simulink model "NDS_FSFB"  (R2022b)
settings: Solver=VariableStepAuto  StartTime=0.0  StopTime=100  RelTol=1e-3
values from neighbouring files (symbols this model uses):
  C_LVLH_ECI0 = [xLVLH__ECI'; yLVLH__ECI'; zLVLH__ECI']    [NDS_FSFBmat.m]
  E_b_LVLH0 = quat2EA(q_b_LVLH0)    [NDS_FSFBmat.m]
  J = [Ixx 0 0 ; 0 Iyy 0; 0 0 Izz]    [NDS_FSFBmat.m]
  kd = 2 .* J * DCR .* w_n    [NDS_FSFBmat.m]
  kp = 2 .* J .* (w_n).^2    [NDS_FSFBmat.m]
  mu = 398600    [ECIstate.m]    (also in NDS_FSFBmat.m)
  n = norm(vECI0)/norm(rECI0)    [NDS_FSFBmat.m]
  q_b_LVLH0 = [eps_LVLH_b0; eta_LVLH_b0]    [NDS_FSFBmat.m]
  q_LVLH_b_c = [0 0 0 1]'    [NDS_FSFBmat.m]
  q_LVLH_ECI0 = C2quat(C_LVLH_ECI0)    [NDS_FSFBmat.m]
  w_ECI_b0_b = w_LVLH_b0_b    [NDS_FSFBmat.m]
undefined symbols (not defined in the file or in its folder): rECI0, vECI0, w_b_ECI0_b
libraries: matrix_library x1
settings Model: Creator=nathaliadesouza  LastModifiedBy=nathaliadesouza
settings DataIOCC: DatasetSignalFormat=timetable

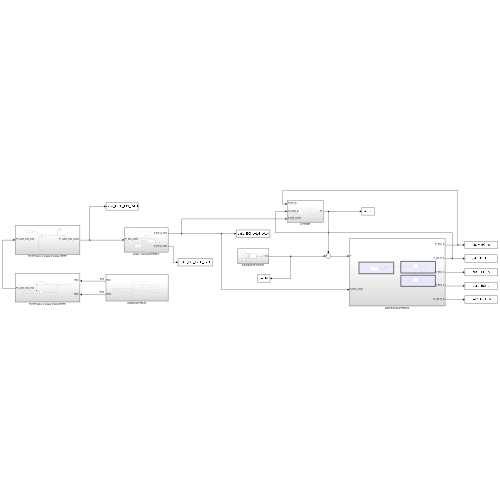
[thumbnail: Simulink's stored preview of the top-level diagram]
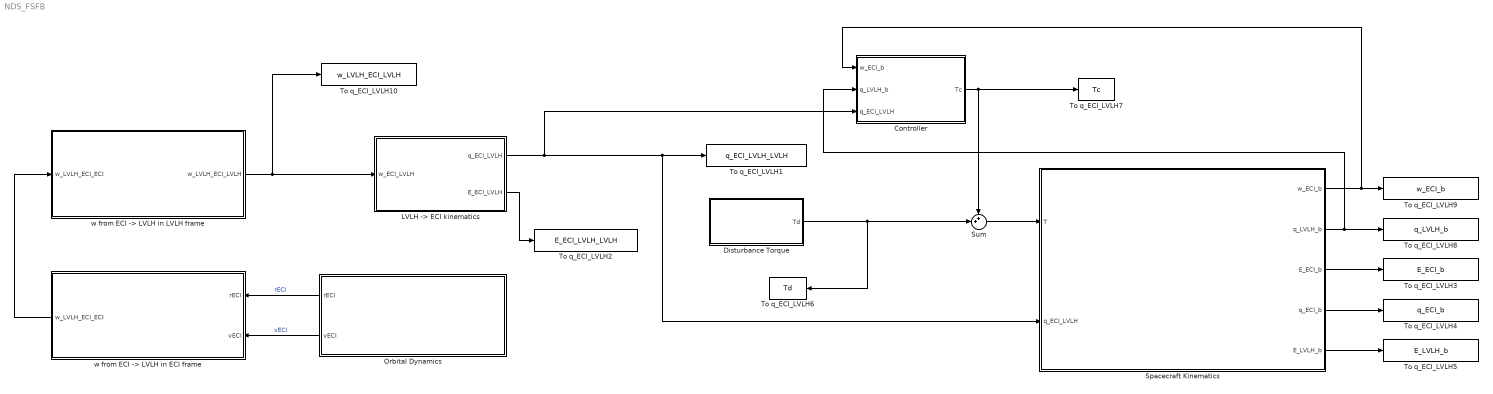
== system NDS_FSFB ==
  Controller : Subsystem
  Disturbance Torque : Subsystem
  "LVLH -> ECI kinematics" : Subsystem
  Orbital Dynamics : Subsystem
  Spacecraft Kinematics : Subsystem
  Sum : Sum  Inputs=++|
  To q_ECI_LVLH1 : ToWorkspace  VariableName=q_ECI_LVLH_LVLH  SaveFormat=Timeseries  SampleTime=-1
  To q_ECI_LVLH10 : ToWorkspace  VariableName=w_LVLH_ECI_LVLH  SaveFormat=Timeseries  SampleTime=-1
  To q_ECI_LVLH2 : ToWorkspace  VariableName=E_ECI_LVLH_LVLH  SaveFormat=Timeseries  SampleTime=-1
  To q_ECI_LVLH3 : ToWorkspace  VariableName=E_ECI_b  SaveFormat=Timeseries  SampleTime=-1
  To q_ECI_LVLH4 : ToWorkspace  VariableName=q_ECI_b  SaveFormat=Timeseries  SampleTime=-1
  To q_ECI_LVLH5 : ToWorkspace  VariableName=E_LVLH_b  SaveFormat=Timeseries  SampleTime=-1
  To q_ECI_LVLH6 : ToWorkspace  VariableName=Td  SaveFormat=Timeseries  SampleTime=-1
  To q_ECI_LVLH7 : ToWorkspace  VariableName=Tc  SaveFormat=Timeseries  SampleTime=-1
  To q_ECI_LVLH8 : ToWorkspace  VariableName=q_LVLH_b  SaveFormat=Timeseries  SampleTime=-1
  To q_ECI_LVLH9 : ToWorkspace  VariableName=w_ECI_b  SaveFormat=Timeseries  SampleTime=-1
  "w from ECI -> LVLH in ECI frame" : Subsystem
  "w from ECI -> LVLH in LVLH frame" : Subsystem
  wires:
  Disturbance Torque/1(Td) -> To q_ECI_LVLH6/1, Sum/2
  "w from ECI -> LVLH in ECI frame"/1(w_LVLH_ECI_ECI) -> "w from ECI -> LVLH in LVLH frame"/1(w_LVLH_ECI_ECI)
  "w from ECI -> LVLH in LVLH frame"/1(w_LVLH_ECI_LVLH) -> To q_ECI_LVLH10/1, "LVLH -> ECI kinematics"/1(w_ECI_LVLH)
  Orbital Dynamics/1(rECI) -> "w from ECI -> LVLH in ECI frame"/1(rECI)  "rECI"
  Orbital Dynamics/2(vECI) -> "w from ECI -> LVLH in ECI frame"/2(vECI)  "vECI"
  "LVLH -> ECI kinematics"/2(E_ECI_LVLH) -> To q_ECI_LVLH2/1
  Sum/1 -> Spacecraft Kinematics/1(T)
  Spacecraft Kinematics/2(q_LVLH_b) -> Controller/2(q_LVLH_b), To q_ECI_LVLH8/1
  Spacecraft Kinematics/1(w_ECI_b) -> Controller/1(w_ECI_b), To q_ECI_LVLH9/1
  Spacecraft Kinematics/3(E_ECI_b) -> To q_ECI_LVLH3/1
  Spacecraft Kinematics/4(q_ECI_b) -> To q_ECI_LVLH4/1
  Spacecraft Kinematics/5(E_LVLH_b) -> To q_ECI_LVLH5/1
  "LVLH -> ECI kinematics"/1(q_ECI_LVLH) -> Spacecraft Kinematics/2(q_ECI_LVLH), To q_ECI_LVLH1/1, Controller/3(q_ECI_LVLH)
  Controller/1(Tc) -> Sum/1, To q_ECI_LVLH7/1

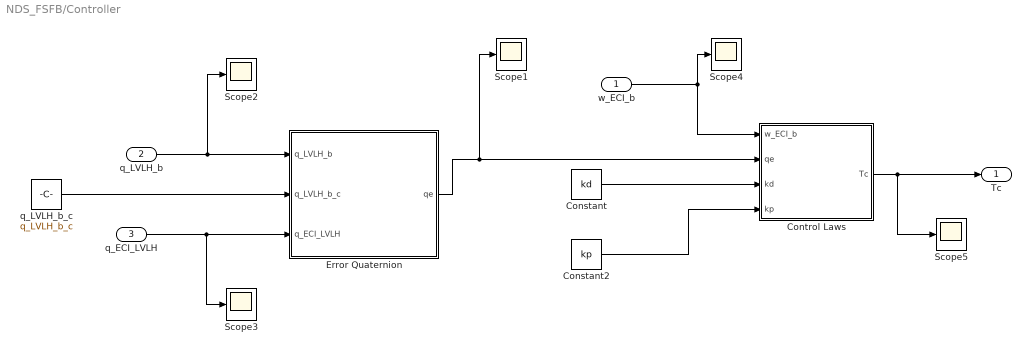
== system NDS_FSFB/Controller ==
  w_ECI_b : Inport
  q_LVLH_b : Inport  Port=2
  q_ECI_LVLH : Inport  Port=3
  Constant : Constant  Value=kd
  Constant2 : Constant  Value=kp
  Control Laws : MATLAB Function  TreatAsAtomicUnit=on
  Error Quaternion : MATLAB Function  TreatAsAtomicUnit=on
  Scope{1..5} (5 alike) : Scope
  q_LVLH_b_c : Constant  Value=q_LVLH_b_c
  Tc : Outport
  wires:
  q_LVLH_b_c/1 -> Error Quaternion/2(q_LVLH_b_c)
  Constant/1 -> Control Laws/3(kd)
  q_LVLH_b/1 -> Scope2/1, Error Quaternion/1(q_LVLH_b)
  q_ECI_LVLH/1 -> Scope3/1, Error Quaternion/3(q_ECI_LVLH)
  Error Quaternion/1(qe) -> Scope1/1, Control Laws/2(qe)
  Constant2/1 -> Control Laws/4(kp)
  w_ECI_b/1 -> Scope4/1, Control Laws/1(w_ECI_b)
  Control Laws/1(Tc) -> Scope5/1, Tc/1

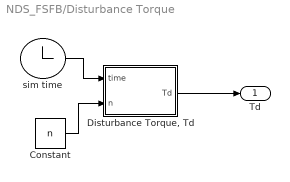
== system NDS_FSFB/Disturbance Torque ==
  Constant : Constant  Value=n
  "Disturbance Torque, Td" : MATLAB Function  TreatAsAtomicUnit=on
  sim time : Clock
  Td : Outport
  wires:
  "Disturbance Torque, Td"/1(Td) -> Td/1
  sim time/1 -> "Disturbance Torque, Td"/1(time)
  Constant/1 -> "Disturbance Torque, Td"/2(n)

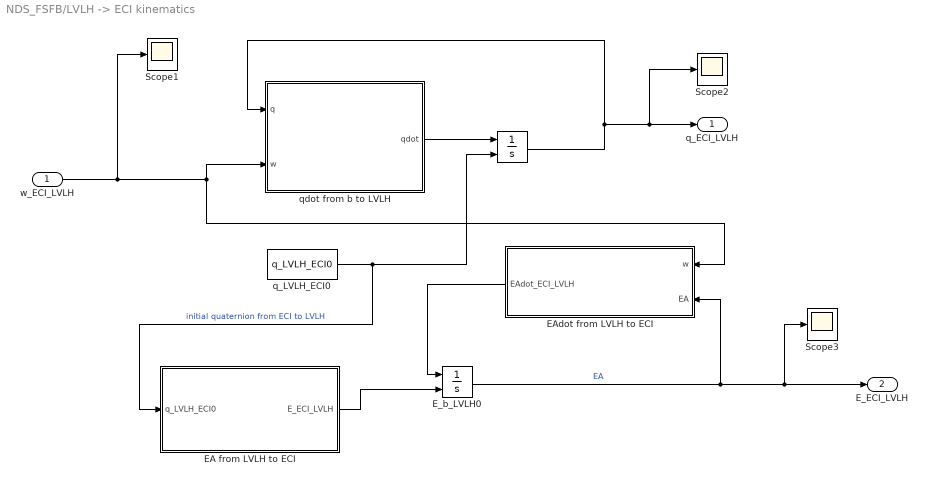
== system NDS_FSFB/LVLH -> ECI kinematics ==
  w_ECI_LVLH : Inport
  " " : Integrator  InitialConditionSource=external  InitialCondition=q_b_LVLH0
  EA from LVLH to ECI : MATLAB Function  TreatAsAtomicUnit=on
  EAdot from LVLH to ECI : MATLAB Function  TreatAsAtomicUnit=on
  E_b_LVLH0 : Integrator  InitialConditionSource=external  InitialCondition=E_b_LVLH0
  Scope1 : Scope
  Scope2 : Scope
  Scope3 : Scope
  q_LVLH_ECI0 : Constant  Value=q_LVLH_ECI0
  qdot from b to LVLH : MATLAB Function  TreatAsAtomicUnit=on
  q_ECI_LVLH : Outport
  E_ECI_LVLH : Outport  Port=2
  wires:
  q_LVLH_ECI0/1 -> EA from LVLH to ECI/1(q_LVLH_ECI0), " "/2  "initial quaternion from ECI to LVLH"
  E_b_LVLH0/1 -> EAdot from LVLH to ECI/2(EA), Scope3/1, E_ECI_LVLH/1  "EA"
  EA from LVLH to ECI/1(E_ECI_LVLH) -> E_b_LVLH0/2
  qdot from b to LVLH/1(qdot) -> " "/1
  w_ECI_LVLH/1 -> Scope1/1, EAdot from LVLH to ECI/1(w), qdot from b to LVLH/2(w)
  EAdot from LVLH to ECI/1(EAdot_ECI_LVLH) -> E_b_LVLH0/1
  " "/1 -> Scope2/1, q_ECI_LVLH/1, qdot from b to LVLH/1(q)

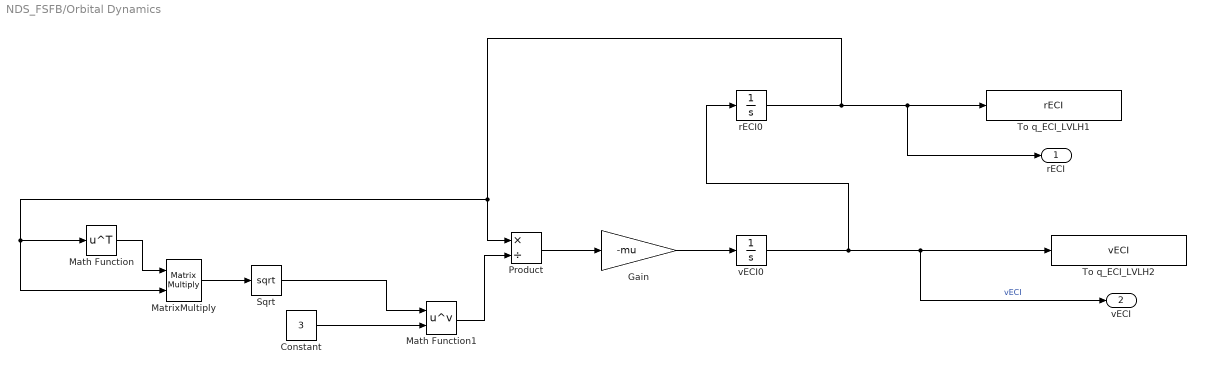
== system NDS_FSFB/Orbital Dynamics ==
  Constant : Constant  Value=3
  Gain : Gain  Gain=-mu
  Math Function : Math  Operator=transpose
  Math Function1 : Math  Operator=pow
  MatrixMultiply : Product  Multiplication=Matrix(*)
  Product : Product  Inputs=*/
  Sqrt : Sqrt
  To q_ECI_LVLH1 : ToWorkspace  VariableName=rECI  SaveFormat=Timeseries  SampleTime=-1
  To q_ECI_LVLH2 : ToWorkspace  VariableName=vECI  SaveFormat=Timeseries  SampleTime=-1
  rECI0 : Integrator  InitialCondition=rECI0
  vECI0 : Integrator  InitialCondition=vECI0
  rECI : Outport
  vECI : Outport  Port=2
  wires:
  Gain/1 -> vECI0/1
  Math Function1/1 -> Product/2
  Constant/1 -> Math Function1/2
  Product/1 -> Gain/1
  rECI0/1 -> rECI/1, To q_ECI_LVLH1/1, MatrixMultiply/2, Math Function/1, Product/1
  MatrixMultiply/1 -> Sqrt/1
  Sqrt/1 -> Math Function1/1
  Math Function/1 -> MatrixMultiply/1
  vECI0/1 -> vECI/1, To q_ECI_LVLH2/1, rECI0/1  "vECI"

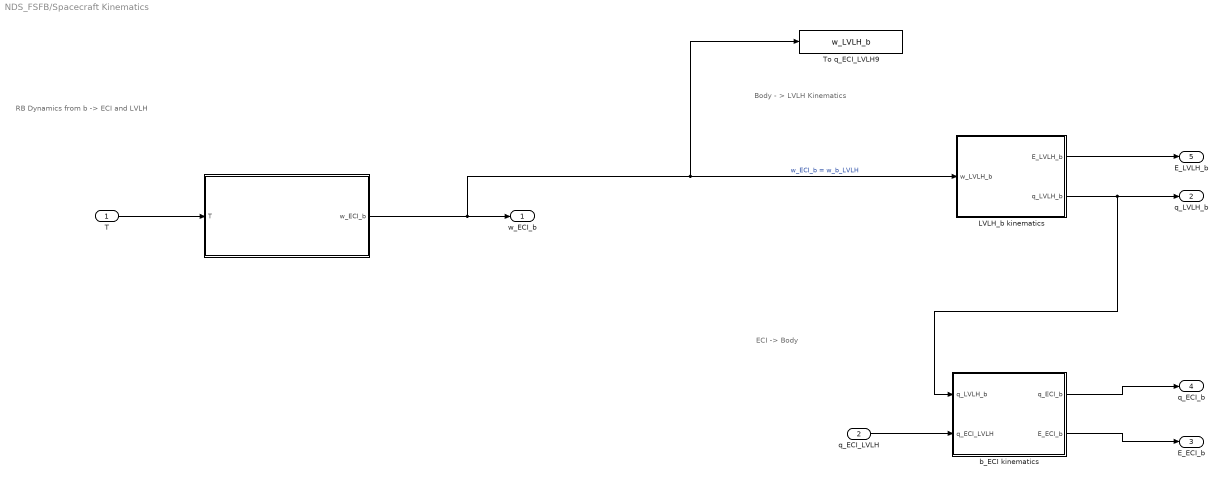
== system NDS_FSFB/Spacecraft Kinematics ==
  note: RB Dynamics from b -> ECI and LVLH
  note: ECI -> Body
  note: Body - > LVLH Kinematics
  T : Inport
  q_ECI_LVLH : Inport  Port=2
  " " : Subsystem
  LVLH_b kinematics : Subsystem
  To q_ECI_LVLH9 : ToWorkspace  VariableName=w_LVLH_b  SaveFormat=Timeseries  SampleTime=-1
  b_ECI kinematics : Subsystem
  w_ECI_b : Outport  PortDimensions=[3 1]
  q_LVLH_b : Outport  Port=2
  E_ECI_b : Outport  Port=3
  q_ECI_b : Outport  Port=4
  E_LVLH_b : Outport  Port=5
  wires:
  b_ECI kinematics/1(q_ECI_b) -> q_ECI_b/1
  b_ECI kinematics/2(E_ECI_b) -> E_ECI_b/1
  LVLH_b kinematics/1(E_LVLH_b) -> E_LVLH_b/1
  LVLH_b kinematics/2(q_LVLH_b) -> b_ECI kinematics/1(q_LVLH_b), q_LVLH_b/1
  T/1 -> " "/1(T)
  " "/1(w_ECI_b) -> w_ECI_b/1, To q_ECI_LVLH9/1, LVLH_b kinematics/1(w_LVLH_b)  "w_ECI_b = w_b_LVLH"
  q_ECI_LVLH/1 -> b_ECI kinematics/2(q_ECI_LVLH)

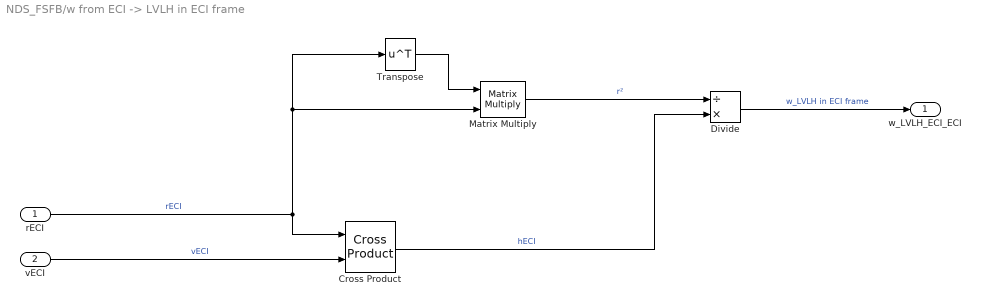
== system NDS_FSFB/w from ECI -> LVLH in ECI frame ==
  rECI : Inport
  vECI : Inport  Port=2
  Cross Product : matrix_library/Cross Product
  Divide : Product  Inputs=/*
  Matrix Multiply : Product  Multiplication=Matrix(*)
  Transpose : Math  Operator=transpose
  w_LVLH_ECI_ECI : Outport
  wires:
  Transpose/1 -> Matrix Multiply/1
  Matrix Multiply/1 -> Divide/1  "r²"
  Cross Product/1 -> Divide/2  "hECI"
  Divide/1 -> w_LVLH_ECI_ECI/1  "w_LVLH in ECI frame"
  rECI/1 -> Matrix Multiply/2, Transpose/1, Cross Product/1  "rECI"
  vECI/1 -> Cross Product/2  "vECI"

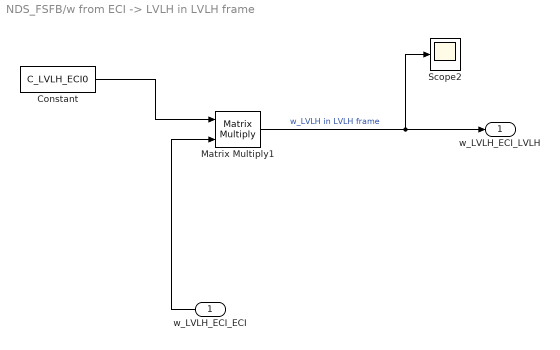
== system NDS_FSFB/w from ECI -> LVLH in LVLH frame ==
  w_LVLH_ECI_ECI : Inport
  Constant : Constant  Value=C_LVLH_ECI0
  Matrix Multiply1 : Product  Multiplication=Matrix(*)
  Scope2 : Scope
  w_LVLH_ECI_LVLH : Outport
  wires:
  Matrix Multiply1/1 -> Scope2/1, w_LVLH_ECI_LVLH/1  "w_LVLH in LVLH frame"
  w_LVLH_ECI_ECI/1 -> Matrix Multiply1/2
  Constant/1 -> Matrix Multiply1/1

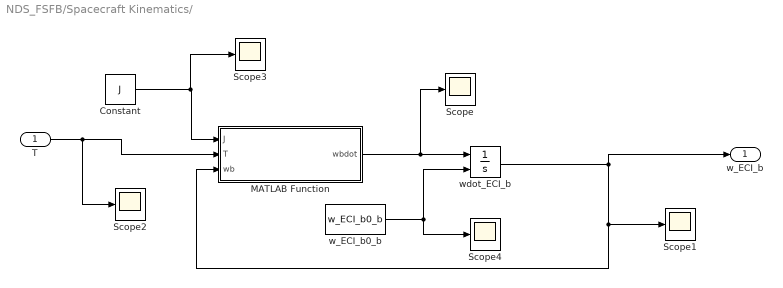
== system NDS_FSFB/Spacecraft Kinematics/  ==
  T : Inport
  Constant : Constant  Value=J
  MATLAB Function : MATLAB Function  TreatAsAtomicUnit=on
  Scope{,1..4} (5 alike) : Scope
  w_ECI_b0_b : Constant  Value=w_ECI_b0_b
  wdot_ECI_b : Integrator  InitialConditionSource=external  InitialCondition=w_b_ECI0_b
  w_ECI_b : Outport  PortDimensions=[3 1]
  wires:
  T/1 -> Scope2/1, MATLAB Function/2(T)
  Constant/1 -> Scope3/1, MATLAB Function/1(J)
  w_ECI_b0_b/1 -> wdot_ECI_b/2, Scope4/1
  wdot_ECI_b/1 -> MATLAB Function/3(wb), Scope1/1, w_ECI_b/1
  MATLAB Function/1(wbdot) -> Scope/1, wdot_ECI_b/1

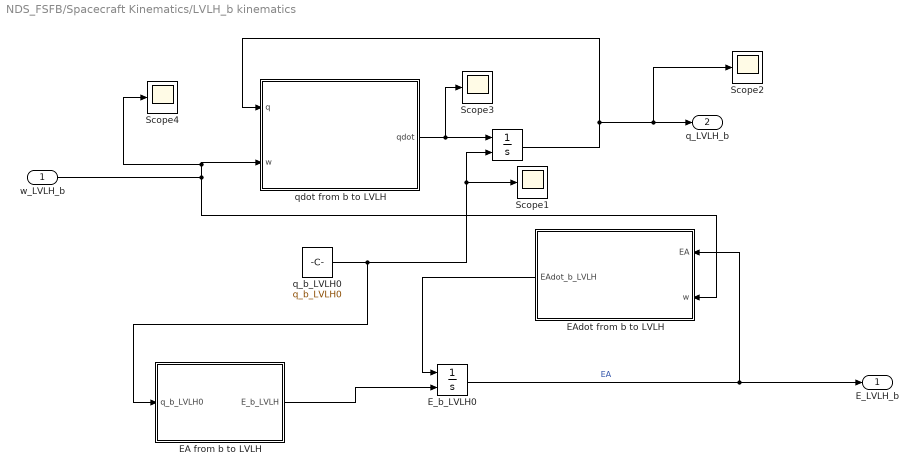
== system NDS_FSFB/Spacecraft Kinematics/LVLH_b kinematics ==
  w_LVLH_b : Inport
  " " : Integrator  InitialConditionSource=external  InitialCondition=q_b_LVLH0
  EA from b to LVLH : MATLAB Function  TreatAsAtomicUnit=on
  EAdot from b to LVLH : MATLAB Function  TreatAsAtomicUnit=on
  E_b_LVLH0 : Integrator  InitialConditionSource=external  InitialCondition=E_b_LVLH0
  Scope{1..4} (4 alike) : Scope
  q_b_LVLH0 : Constant  Value=q_b_LVLH0
  qdot from b to LVLH : MATLAB Function  TreatAsAtomicUnit=on
  E_LVLH_b : Outport
  q_LVLH_b : Outport  Port=2
  wires:
  q_b_LVLH0/1 -> EA from b to LVLH/1(q_b_LVLH0), Scope1/1, " "/2
  E_b_LVLH0/1 -> EAdot from b to LVLH/1(EA), E_LVLH_b/1  "EA"
  EA from b to LVLH/1(E_b_LVLH) -> E_b_LVLH0/2
  qdot from b to LVLH/1(qdot) -> Scope3/1, " "/1
  w_LVLH_b/1 -> Scope4/1, qdot from b to LVLH/2(w), EAdot from b to LVLH/2(w)
  EAdot from b to LVLH/1(EAdot_b_LVLH) -> E_b_LVLH0/1
  " "/1 -> Scope2/1, q_LVLH_b/1, qdot from b to LVLH/1(q)

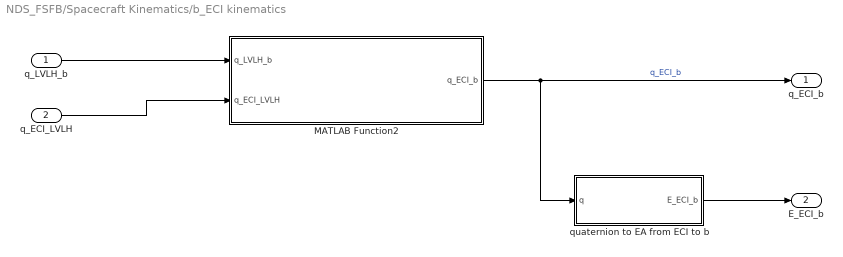
== system NDS_FSFB/Spacecraft Kinematics/b_ECI kinematics ==
  q_LVLH_b : Inport
  q_ECI_LVLH : Inport  Port=2
  MATLAB Function2 : MATLAB Function  TreatAsAtomicUnit=on
  quaternion to EA from ECI to b : MATLAB Function  TreatAsAtomicUnit=on
  q_ECI_b : Outport
  E_ECI_b : Outport  Port=2
  wires:
  quaternion to EA from ECI to b/1(E_ECI_b) -> E_ECI_b/1
  q_LVLH_b/1 -> MATLAB Function2/1(q_LVLH_b)
  MATLAB Function2/1(q_ECI_b) -> q_ECI_b/1, quaternion to EA from ECI to b/1(q)  "q_ECI_b"
  q_ECI_LVLH/1 -> MATLAB Function2/2(q_ECI_LVLH)

== matlab function NDS_FSFB/Spacecraft Kinematics/ /MATLAB Function ==
  data: J input; wbdot output; T input; wb input
function wbdot = eulereqn(J, T, wb)

wbdot = inv(J) * (T - crossvect(wb) * J * wb);

end

== matlab function NDS_FSFB/Spacecraft Kinematics/b_ECI kinematics/quaternion to EA from ECI to b ==
  data: q input; E_ECI_b output
function E_ECI_b = quat2EA(q)

eta = q(4);
eps = q(1:3);
    
phi = atan2(2 * (eta * eps(1) + eps(2) * eps(3)), 1 - 2 * (eps(1)^2 + eps(2)^2));

if (2 * (eta * eps(2) - eps(3) * eps(1)) >= 1 | 2 * (eta * eps(2) - eps(3) * eps(1)) <= -1)
    theta = 0;
else
    theta = asin(2 * (eta * eps(2) - eps(3) * eps(1)));
end


psi = atan2(2 * (eta * eps(3) + eps(1) * eps(2)), 1 - 2 * (eps(2)^2 + eps(3)^2)) - pi/2;
    
E_ECI_b = [phi theta psi]';

end

== matlab function NDS_FSFB/LVLH -> ECI kinematics/EA from LVLH to ECI ==
  data: q_LVLH_ECI0 input; E_ECI_LVLH output
function E_ECI_LVLH  = EALVLHtoECI(q_LVLH_ECI0)

E_ECI_LVLH = quat2EA(q_LVLH_ECI0);

end

== matlab function NDS_FSFB/Disturbance Torque/Disturbance Torque, Td ==
  data: time input; Td output; n input
function Td = Td(time, n)

Td = 10^-3 .* sin(3 * n * time) .* [0; 0.5; 0]; % [N * m]

end

== matlab function NDS_FSFB/Controller/Error Quaternion ==
  data: q_LVLH_b input; q_LVLH_b_c input; qe output; q_ECI_LVLH input
function qe = quaterror(q_LVLH_b, q_LVLH_b_c, q_ECI_LVLH)

q_ECI_b = quatmult(quatconj(q_ECI_LVLH), q_LVLH_b);
q_ECI_b_c = quatmult(quatconj(q_ECI_LVLH), q_LVLH_b_c); % target quaternion

qe = quatmult(quatconj(q_ECI_b_c), q_ECI_b);

end

== matlab function NDS_FSFB/LVLH -> ECI kinematics/EAdot from LVLH to ECI ==
  data: w input; EA input; EAdot_ECI_LVLH output
function EAdot_ECI_LVLH = EAdot(w,EA)

% Euler angle differentiation equation
phi = EA(1);
theta = EA(2);
psi = EA(3);

EAdot_ECI_LVLH = [cos(theta), sin(phi) * sin(theta), cos(phi) * sin(theta); ...
        0, cos(phi) * cos(theta), -sin(phi) * cos(theta); ...
        0, sin(phi), cos(phi)] / cos(theta) * w;

end

== matlab function NDS_FSFB/LVLH -> ECI kinematics/qdot from b to LVLH ==
  data: q input; qdot output; w input
function qdot = quatdiff(q, w)

% qdot = quatdiff(q_ECI_LVLH, w_ECI_LVLH);

% quaternion differentiation equation
epsX = [0 -q(3) q(2); q(3) 0 -q(1); -q(2) q(1) 0];


eta = q(4);
e = q(1:3);

dot_eta = -e' * w / 2;
dot_e = (eta * eye(3) + epsX) * w / 2;

qdot = [dot_e; dot_eta];



end

== matlab function NDS_FSFB/Spacecraft Kinematics/LVLH_b kinematics/EA from b to LVLH ==
  data: q_b_LVLH0 input; E_b_LVLH output
function E_b_LVLH  = EALVLHtob(q_b_LVLH0)

E_b_LVLH = quat2EA(q_b_LVLH0);

end

== matlab function NDS_FSFB/Controller/Control Laws ==
  data: w_ECI_b input; qe input; Tc output; kd input; kp input
function Tc = Tctrl(w_ECI_b, qe, kd, kp)


etae = qe(4);
epse = qe(1:3);

Tc = (-kp .* sign(etae) * epse) - (kd * w_ECI_b); % part A
% Tc = (-sign(etae) .* kp * epse) - kd * (1 - transpose(etae) * etae) * w_ECI_b; % part B
% Tc = (-sign(etae) .* kp * epse) - kd * (1 + transpose(etae) * etae) * w_ECI_b; % part C

end

== matlab function NDS_FSFB/Spacecraft Kinematics/LVLH_b kinematics/EAdot from b to LVLH ==
  data: EA input; EAdot_b_LVLH output; w input
function EAdot_b_LVLH = EAdot(EA, w)

% Euler angle differentiation equation
phi = EA(1);
theta = EA(2);
psi = EA(3);

EAdot_b_LVLH = [cos(theta), sin(phi) * sin(theta), cos(phi) * sin(theta); ...
        0, cos(phi) * cos(theta), -sin(phi) * cos(theta); ...
        0, sin(phi), cos(phi)] / cos(theta) * w;

end

== matlab function NDS_FSFB/Spacecraft Kinematics/LVLH_b kinematics/qdot from b to LVLH ==
  data: q input; qdot output; w input
function qdot = qdot_LVLH_b(q, w)

%qdot = quatdiff(q_LVLH_b, w_b_LVLH);


eta = q(4);
eps = q(1:3);

etadot = -eps' * w / 2;
epsdot = (eta * eye(3) + crossvect(eps)) * w / 2;

qdot = [epsdot; etadot];

end

== matlab function NDS_FSFB/Spacecraft Kinematics/b_ECI kinematics/MATLAB Function2 ==
  data: q_LVLH_b input; q_ECI_b output; q_ECI_LVLH input
function q_ECI_b  = qLVLHtoECI(q_LVLH_b, q_ECI_LVLH)

q_ECI_b = quatmult(q_ECI_LVLH, q_LVLH_b);

end
